simulink model "VikulovTask1"  (Simulink 7.8)
settings: Solver=ode45  StartTime=0.0  StopTime=10.0  RelTol=1e-3
libraries: simulink x3
settings Model: Creator=--  LastModifiedBy=--

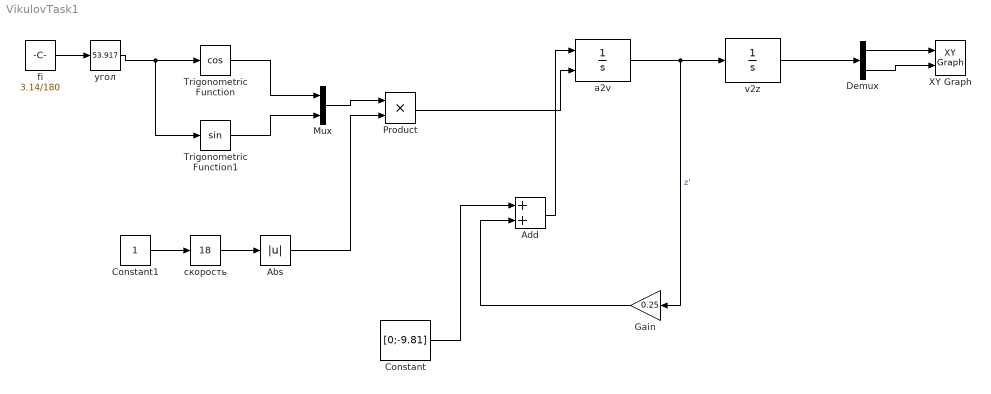
== system VikulovTask1 ==
  Abs : Abs
  Add : Sum
  Constant : Constant  Value=[0;-9.81]
  Constant1 : Constant
  Demux : Demux  Outputs=2
  Gain : Gain  Gain=0.25
  Mux : Mux  Inputs=2
  Product : Product  RndMeth=Zero
  Trigonometric Function : Trigonometry  Operator=cos
  Trigonometric Function1 : Trigonometry
  XY Graph : simulink/Sinks/XY Graph  xmin=0  xmax=100  ymin=0  ymax=30  st=-1
  a2v : Integrator  InitialConditionSource=external  InitialCondition=[10;10]  UpperSaturationLimit=1  LowerSaturationLimit=0
  fi : Constant  Value=3.14/180
  v2z : Integrator  UpperSaturationLimit=1  LowerSaturationLimit=0
  скорость : simulink/Math Operations/Slider Gain  low=0  gain=18  high=100
  угол : simulink/Math Operations/Slider Gain  low=0  gain=53.917  high=90
  wires:
  a2v/1 -> v2z/1, Gain/1  "z'"
  Gain/1 -> Add/2
  Constant/1 -> Add/1
  Add/1 -> a2v/1
  v2z/1 -> Demux/1
  Demux/1 -> XY Graph/1
  Demux/2 -> XY Graph/2
  fi/1 -> угол/1
  Trigonometric Function/1 -> Mux/1
  Trigonometric Function1/1 -> Mux/2
  Mux/1 -> Product/1
  Abs/1 -> Product/2
  Product/1 -> a2v/2
  угол/1 -> Trigonometric Function/1, Trigonometric Function1/1
  Constant1/1 -> скорость/1
  скорость/1 -> Abs/1
